simulink model "Controllo_SS_Template_2019b"  (R2019b)
settings: Solver=VariableStepAuto  StartTime=0.0  StopTime=10.0  RelTol=1e-3
values from neighbouring files (symbols this model uses):
  A_ob = A - L_kf*C    [LQ_KF.m]    (also in LQ_KF_version1.m; LQ_KF_version2.m; LQ_Luenberger.m = A - L*C; LQ_prova.m)
  B_ob = [ B - L_kf*D, L_kf]    [LQ_KF.m]    (also in LQ_KF_version1.m; LQ_KF_version2.m; LQ_Luenberger.m = [ B - L*D, L]; LQ_prova.m)
  C_ob = eye(n)    [LQ_KF.m]    (also in LQ_KF_version1.m; LQ_KF_version2.m; LQ_Luenberger.m; LQ_prova.m)
  D_ob = zeros(n, m+p)    [LQ_KF.m]    (also in LQ_KF_version1.m; LQ_KF_version2.m; LQ_Luenberger.m; LQ_prova.m)
  Ken_eta = K(:, 4)    [LQ_KF.m]    (also in LQ_KF_version1.m; LQ_KF_version2.m = Ken(:, n+1:end); LQ_Luenberger.m; LQ_prova.m = Ken(:, n+1:end))
  Ken_x = K(:, 1:3)    [LQ_KF.m]    (also in LQ_KF_version1.m; LQ_KF_version2.m = Ken(:, 1:n); LQ_Luenberger.m; LQ_prova.m = Ken(:, 1:n))
  Lower_bound_V = 0    [LQ_KF.m]    (also in LQ_KF_version1.m; LQ_KF_version2.m; LQ_Luenberger.m; LQ_prova.m)
  Upper_bound_V = 23    [LQ_KF.m]    (also in LQ_KF_version1.m; LQ_KF_version2.m; LQ_Luenberger.m; LQ_prova.m)
undefined symbols (not defined in the file or in its folder): HIL, Kb, offset_corrente_volt, offset_posizione_volt, x1_eq0, x2_eq0
libraries: quarc_library x4, simulink x1
settings Model: Creator=Pronto all'uso  LastModifiedBy=Student
settings DebuggingCC: UnconnectedInputMsg=none  UnconnectedOutputMsg=none  UnconnectedLineMsg=none
settings ModelReferenceCC: EnableRefExpFcnMdlSchedulingChecks=off
settings RTWCC: Description=Generic Real-Time Target

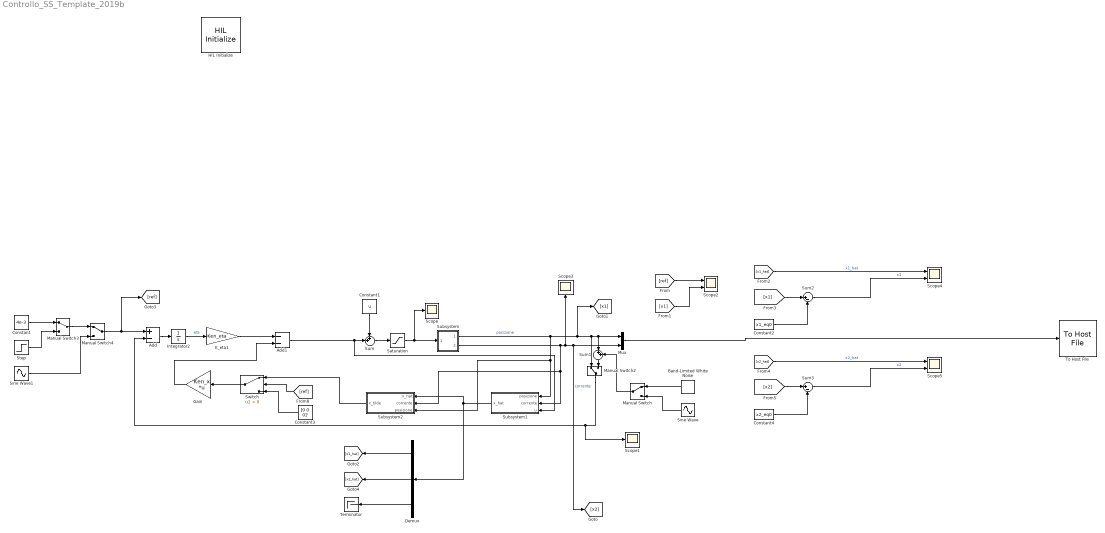
== system Controllo_SS_Template_2019b ==
  Add : Sum  Inputs=+-
  Add1 : Sum  Inputs=--
  Band-Limited White Noise : simulink/Sources/Band-Limited White Noise  Cov=[8.9934e-11*0.002]  Ts=0.002  seed=[23341]
  Constant : Constant  Value=4e-3
  Constant1 : Constant  Value=u
  Constant2 : Constant  Value=x1_eq0
  Constant3 : Constant  Value=[0 0 0]'
  Constant4 : Constant  Value=x2_eq0
  Demux : Demux  Outputs=3
  Gain : Gain  Gain=Ken_x  Multiplication=Matrix(K*u) (u vector)
  HIL Initialize : quarc_library/Data Acquisition/Generic/Configuration/HIL Initialize  Priority=-99  object_name=HIL-1  board_type=q2_usb  board_number=0  board_options=d0=digital;d1=digital;led=auto;update_rate=normal;decimation=1  exclusive=off  active=off  hardware_clocks=[0]  clock_modes=[]  initial_clock_frequencies=[]  set_clock_params_at_start=off  set_clock_params_at_switch_in=off  set_clock_frequencies_at_start=off  set_clock_frequencies_at_switch_in=off  analog_input_channels=[0:1]  analog_input_configurations=[]  analog_input_maximums=10  analog_input_minimums=-10  set_analog_input_params_at_start=on  set_analog_input_params_at_switch_in=off  analog_output_channels=[0:1]  analog_output_maximums=10  analog_output_minimums=-10  initial_analog_outputs=[0]  final_analog_outputs=[0]  watchdog_analog_outputs=0  set_analog_output_params_at_start=on  set_analog_output_params_at_switch_in=off  set_analog_outputs_at_start=on  set_analog_outputs_at_switch_in=off  set_analog_outputs_at_terminate=on  set_analog_outputs_at_switch_out=off  set_analog_outputs_on_watchdog=off  digital_input_channels=[]  digital_output_channels=[]  digital_output_configuration=[]  initial_digital_outputs=[1]  final_digital_outputs=[1]  watchdog_digital_outputs=[1]  set_digital_output_params_at_start=off  set_digital_output_params_at_switch_in=off  set_digital_outputs_at_start=on  set_digital_outputs_at_switch_in=off  set_digital_outputs_at_terminate=on  set_digital_outputs_at_switch_out=off  set_digital_outputs_on_watchdog=off  encoder_channels=[0:1]  quadrature=[4]  encoder_filter_frequency=[]  initial_encoder_counts=[0]  set_encoder_params_at_start=on  set_encoder_params_at_switch_in=off  set_encoder_counts_at_start=on  set_encoder_counts_at_switch_in=off  pwm_channels=[]  pwm_modes=[0]  pwm_frequency=1/0.020  pwm_configuration=[]  pwm_alignment=[]  pwm_polarity=[]  pwm_leading_deadband=[]  pwm_trailing_deadband=[]  initial_pwm_outputs=[0]  final_pwm_outputs=[0]  watchdog_pwm_outputs=[0]  set_pwm_params_at_start=on  set_pwm_params_at_switch_in=off  set_pwm_outputs_at_start=on  set_pwm_outputs_at_switch_in=off  set_pwm_outputs_at_terminate=on  set_pwm_outputs_at_switch_out=off  set_pwm_outputs_on_watchdog=off  other_output_channels=[]  initial_other_outputs=[]  final_other_outputs=[]  watchdog_other_outputs=[]  set_other_outputs_at_start=off  set_other_outputs_at_switch_in=off  set_other_outputs_at_terminate=off  set_other_outputs_at_switch_out=off  set_other_outputs_on_watchdog=off
  Integrator2 : Integrator
  K_eta1 : Gain  Gain=Ken_eta
  Manual Switch{,2..4} (4 alike) : ManualSwitch
  Mux : Mux  Inputs=2
  Saturation : Saturate  UpperLimit=Upper_bound_V  LowerLimit=Lower_bound_V
  Scope : Scope
  Scope1 : Scope
  Scope2 : Scope  NumInputPorts=2
  Scope3 : Scope
  Scope4 : Scope  NumInputPorts=2
  Scope5 : Scope  NumInputPorts=2
  Sine Wave : Sin  SampleTime=0
  Sine Wave1 : Sin  SampleTime=0
  Step : Step  Time=2  After=0.003  SampleTime=0
  Subsystem : Subsystem
  Subsystem1 : Subsystem
  Subsystem2 : Subsystem
  Sum : Sum  Inputs=++|
  Sum1 : Sum  Inputs=|++
  Sum2 : Sum  Inputs=|+-
  Sum3 : Sum  Inputs=|+-
  Switch : Switch  Criteria=u2 > Threshold
  Terminator : Terminator
  To Host File : quarc_library/Sinks/To Host/To Host File  file_name=data_%{date}_%{time}.mat  variable_name=data_%{date}_%{time}  decimation=1  sample_time=-1  file_format=MAT-file v.5  options=No header or footer  append=off  final_file_name=data_13-May-2025_17-04-53.mat  bitrate=2000000
  wires:
  [x1] -> Scope2/2
  Mux/1 -> To Host File/1
  Manual Switch/1 -> Sum1/2
  K_eta1/1 -> Add1/1
  Constant/1 -> Manual Switch3/1
  Sine Wave/1 -> Manual Switch/2
  Band-Limited White Noise/1 -> Manual Switch/1
  Manual Switch3/1 -> Manual Switch4/1
  Subsystem/2(Input) -> Subsystem2/2(corrente), Subsystem1/2(corrente), Scope3/1, Mux/2, [x2]  "corrente"
  Manual Switch2/1 -> Add/2, Scope1/1
  Add/1 -> Integrator2/1
  Sum/1 -> Saturation/1
  [ref] -> Scope2/1
  Constant1/1 -> Sum/1
  Step/1 -> Manual Switch3/2
  Integrator2/1 -> K_eta1/1  "eta"
  Sine Wave1/1 -> Manual Switch4/2
  Add1/1 -> Subsystem1/3(u), Sum/2
  Subsystem/1(posizione) -> [x1], Manual Switch2/1, Mux/1, Sum1/1, Subsystem2/3(posizione), Subsystem1/1(posizione)  "posizione"
  Sum1/1 -> Manual Switch2/2
  Manual Switch4/1 -> Add/1, [ref]
  Saturation/1 -> Scope/1, Subsystem/1(In1)
  Constant3/1 -> Switch/3
  [ref] -> Switch/2
  Switch/1 -> Gain/1
  Subsystem1/1(x_hat) -> Subsystem2/1(x_hat), Demux/1
  Gain/1 -> Add1/2
  Demux/2 -> [x2_hat]
  Demux/1 -> [x1_hat]
  [x2_hat] -> Scope5/1  "x2_hat"
  Constant4/1 -> Sum3/2
  Sum3/1 -> Scope5/2  "x2"
  [x1] -> Sum2/1
  Sum2/1 -> Scope4/2  "x1"
  [x1_hat] -> Scope4/1  "x1_hat"
  Constant2/1 -> Sum2/2
  [x2] -> Sum3/1
  Subsystem2/1(x_tilde) -> Switch/1
  Demux/3 -> Terminator/1

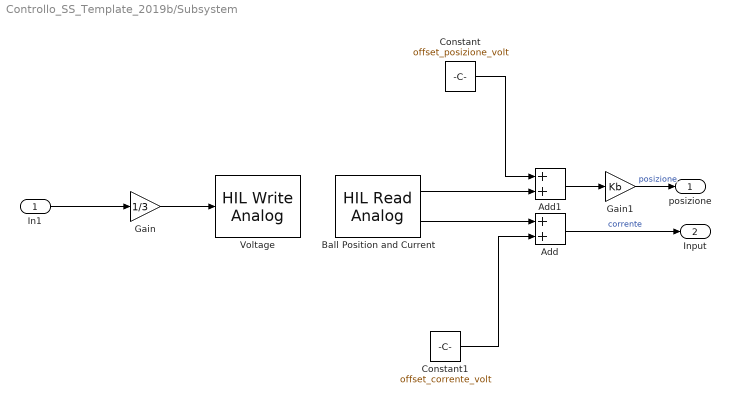
== system Controllo_SS_Template_2019b/Subsystem ==
  In1 : Inport
  Add : Sum
  Add1 : Sum
  Ball Position and Current : quarc_library/Data Acquisition/Generic/Immediate I//O/HIL Read Analog  object_name=HIL-1  channels=[0:1]  sample_time=qc_get_step_size  active=on  vector_output=off
  Constant : Constant  Value=offset_posizione_volt
  Constant1 : Constant  Value=offset_corrente_volt
  Gain : Gain  Gain=1/3
  Gain1 : Gain  Gain=Kb
  Voltage : quarc_library/Data Acquisition/Generic/Immediate I//O/HIL Write Analog  object_name=HIL-1  channels=0  sample_time=-1  active=off  vector_input=off
  posizione : Outport
  Input : Outport  Port=2
  wires:
  Ball Position and Current/1 -> Add1/2
  In1/1 -> Gain/1
  Ball Position and Current/2 -> Add/1
  Gain/1 -> Voltage/1
  Gain1/1 -> posizione/1  "posizione"
  Add1/1 -> Gain1/1
  Add/1 -> Input/1  "corrente"
  Constant1/1 -> Add/2
  Constant/1 -> Add1/1

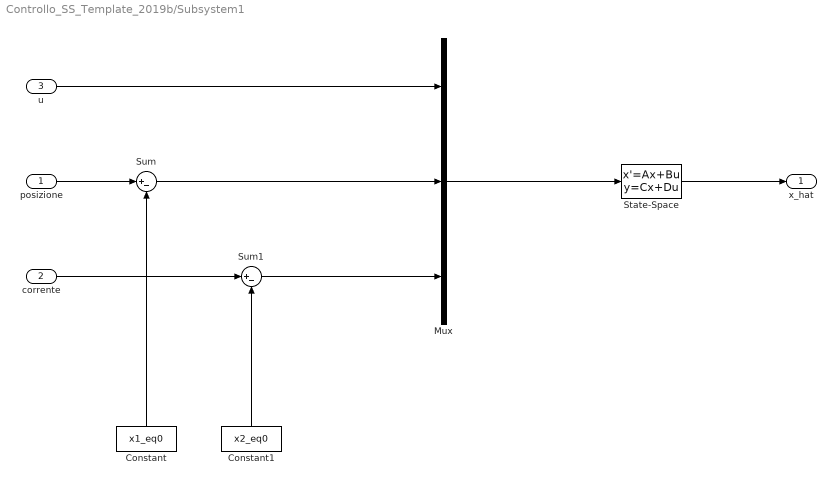
== system Controllo_SS_Template_2019b/Subsystem1 ==
  posizione : Inport
  corrente : Inport  Port=2
  u : Inport  Port=3
  Constant : Constant  Value=x1_eq0
  Constant1 : Constant  Value=x2_eq0
  Mux : Mux  Inputs=3
  State-Space : StateSpace  A=A_ob  B=B_ob  C=C_ob  D=D_ob  InitialCondition=[-x1_eq0, -x2_eq0, 0]
  Sum : Sum  Inputs=|+-
  Sum1 : Sum  Inputs=|+-
  x_hat : Outport
  wires:
  posizione/1 -> Sum/1
  Constant/1 -> Sum/2
  Constant1/1 -> Sum1/2
  corrente/1 -> Sum1/1
  u/1 -> Mux/1
  Sum/1 -> Mux/2
  Sum1/1 -> Mux/3
  State-Space/1 -> x_hat/1
  Mux/1 -> State-Space/1

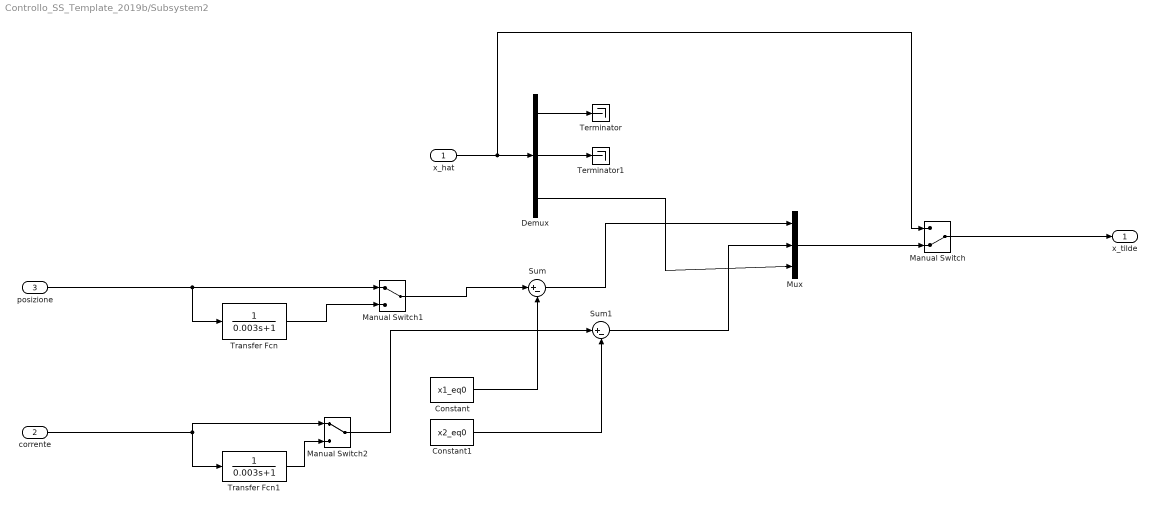
== system Controllo_SS_Template_2019b/Subsystem2 ==
  x_hat : Inport
  corrente : Inport  Port=2
  posizione : Inport  Port=3
  Constant : Constant  Value=x1_eq0
  Constant1 : Constant  Value=x2_eq0
  Demux : Demux  Outputs=3
  Manual Switch : ManualSwitch  CurrentSetting=0
  Manual Switch1 : ManualSwitch
  Manual Switch2 : ManualSwitch
  Mux : Mux  Inputs=3
  Sum : Sum  Inputs=|+-
  Sum1 : Sum  Inputs=|+-
  Terminator : Terminator
  Terminator1 : Terminator
  Transfer Fcn : TransferFcn  Denominator=[0.003 1]
  Transfer Fcn1 : TransferFcn  Denominator=[0.003 1]
  x_tilde : Outport
  wires:
  x_hat/1 -> Manual Switch/1, Demux/1
  Manual Switch/1 -> x_tilde/1
  Demux/1 -> Terminator/1
  Demux/2 -> Terminator1/1
  Mux/1 -> Manual Switch/2
  Demux/3 -> Mux/3
  Sum/1 -> Mux/1
  Sum1/1 -> Mux/2
  Constant/1 -> Sum/2
  Constant1/1 -> Sum1/2
  posizione/1 -> Transfer Fcn/1, Manual Switch1/1
  Manual Switch1/1 -> Sum/1
  Transfer Fcn/1 -> Manual Switch1/2
  corrente/1 -> Transfer Fcn1/1, Manual Switch2/1
  Manual Switch2/1 -> Sum1/1
  Transfer Fcn1/1 -> Manual Switch2/2
